simulink model "PID_model_system_creation"  (R2023a)
settings: Solver=VariableStepAuto  StartTime=0.0  StopTime=10.0  RelTol=1e-3
undefined symbols (not defined in the file or in its folder): K_p, Kd, Ki, Ts
settings Model: Creator=mazen  LastModifiedBy=mazen

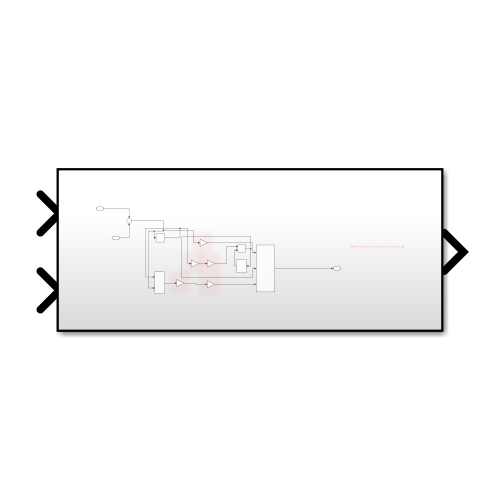
[thumbnail: Simulink's stored preview of the top-level diagram]
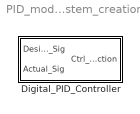
== system PID_model_system_creation ==
  Digital_PID_Controller : Subsystem

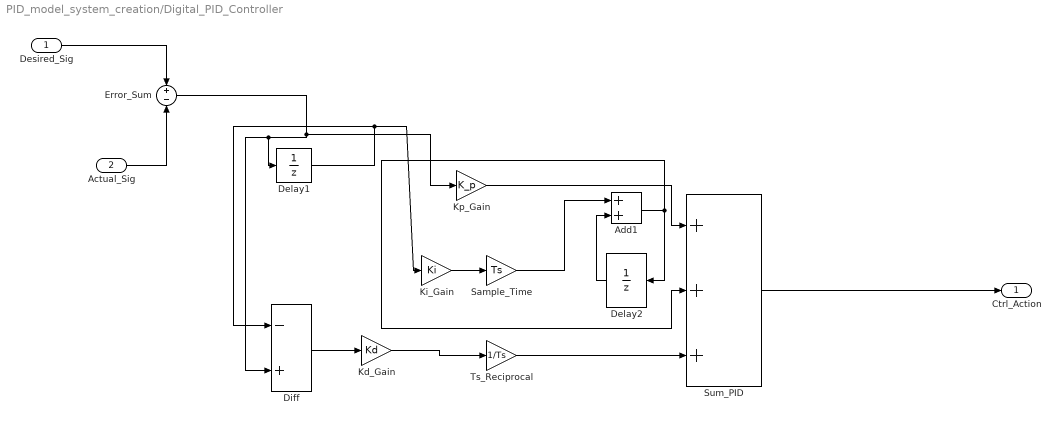
== system PID_model_system_creation/Digital_PID_Controller ==
  Desired_Sig : Inport
  Actual_Sig : Inport  Port=2
  Add1 : Sum
  Delay1 : UnitDelay  SampleTime=-1  HasFrameUpgradeWarning=on
  Delay2 : UnitDelay  SampleTime=-1  HasFrameUpgradeWarning=on
  Diff : Sum  Inputs=-+
  Error_Sum : Sum  Inputs=+-
  Kd_Gain : Gain  Gain=Kd
  Ki_Gain : Gain  Gain=Ki
  Kp_Gain : Gain  Gain=K_p
  Sample_Time : Gain  Gain=Ts
  Sum_PID : Sum  Inputs=+++
  Ts_Reciprocal : Gain  Gain=1/Ts
  Ctrl_Action : Outport
  wires:
  ? -> ?
  Desired_Sig/1 -> Error_Sum/1
  Actual_Sig/1 -> Error_Sum/2
  Error_Sum/1 -> Delay1/1, Diff/2, Kp_Gain/1
  Kp_Gain/1 -> Sum_PID/1
  Delay1/1 -> Diff/1, Ki_Gain/1
  Ki_Gain/1 -> Sample_Time/1
  Sample_Time/1 -> Add1/1
  Add1/1 -> Delay2/1, Sum_PID/2
  Delay2/1 -> Add1/2
  Diff/1 -> Kd_Gain/1
  Kd_Gain/1 -> Ts_Reciprocal/1
  Ts_Reciprocal/1 -> Sum_PID/3
  Sum_PID/1 -> Ctrl_Action/1
